simulink model "Simulation_traj"  (R2023a)
settings: Solver=FixedStepAuto  StartTime=0.0  StopTime=30  FixedStep=0.001  RelTol=1e-1
settings Model: Creator=mattia  LastModifiedBy=mattia
settings OptimizationCC: BlockReduction=off  DefaultParameterBehavior=Inlined  BufferReuse=off

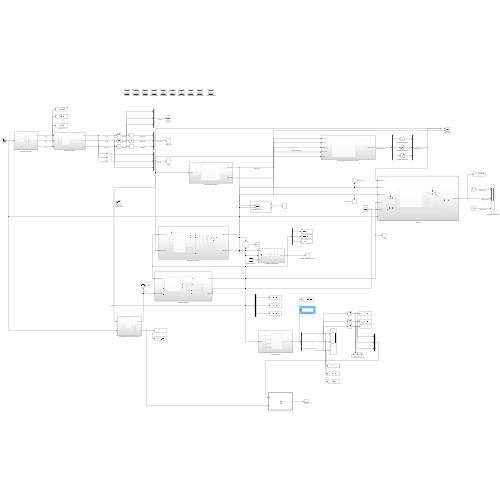
[thumbnail: Simulink's stored preview of the top-level diagram]
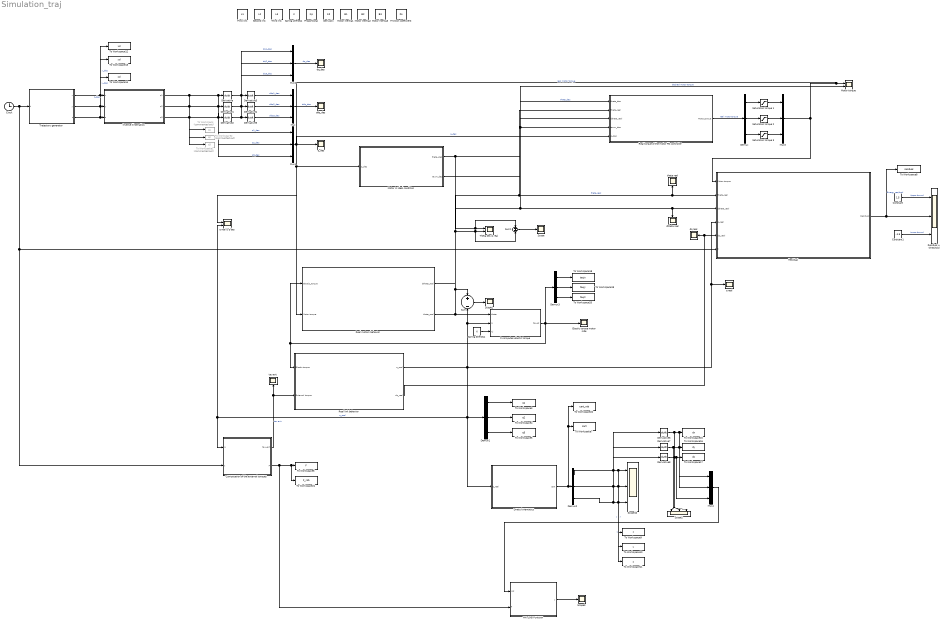
== system Simulation_traj ==
  Clock : Clock
  Computation of the external torques : Subsystem
  Constant : Constant  Value=1.5
  Constant1 : Constant  Value=-1.5
  Demux{,1..3} (4 alike) : Demux  Outputs=3
  Derivativ : DataStoreMemory  DataStoreName=Kd  WriteAfterWriteMsg=warning  InitialValue=50  ShowAdditionalParam=off
  Derivative{,1..8} (9 alike) : Derivative
  Direct kinematics : Subsystem
  Elastic torque motor side : Scope
  FIrst link : DataStoreMemory  DataStoreName=L1  WriteAfterWriteMsg=warning  InitialValue=0.5  ShowAdditionalParam=off
  Friction coefficient : DataStoreMemory  DataStoreName=Dv  WriteAfterWriteMsg=warning  InitialValue=0.8  ShowAdditionalParam=off
  Inverse Kinematics : Subsystem
  It computes elastic torque : Subsystem
  MATLAB Function : MATLAB Function  TreatAsAtomicUnit=on
  Motor Inertia1 : DataStoreMemory  DataStoreName=B1  WriteAfterWriteMsg=warning  InitialValue=0.45  ShowAdditionalParam=off
  Motor Inertia2 : DataStoreMemory  DataStoreName=B2  WriteAfterWriteMsg=warning  InitialValue=0.3037  ShowAdditionalParam=off
  Motor Inertia3 : DataStoreMemory  DataStoreName=B3  WriteAfterWriteMsg=warning  InitialValue=0.1199  ShowAdditionalParam=off
  Motor in ideal condition : Subsystem
  Motor torque : Scope  NumInputPorts=2
  Mux{,1..4} (5 alike) : Mux  Inputs=3
  Proportional : DataStoreMemory  DataStoreName=Kp  WriteAfterWriteMsg=warning  InitialValue=150  ShowAdditionalParam=off
  Real link behavior : Subsystem
  Real motors behavior : Subsystem
  Real torque of the motor PD controller : Subsystem
  Residual : Subsystem
  Residual + threshold : Scope  NumInputPorts=3
  Saturation torque 1 : Saturate  UpperLimit=80  LowerLimit=-80
  Saturation torque 2 : Saturate  UpperLimit=80  LowerLimit=-80
  Saturation torque 3 : Saturate  UpperLimit=80  LowerLimit=-80
  Scope : Scope
  Scope1 : Scope
  Scope10 : Scope  NumInputPorts=3
  Scope2 : Scope  NumInputPorts=3
  Scope3 : Scope
  Second link : DataStoreMemory  DataStoreName=L2  WriteAfterWriteMsg=warning  InitialValue=0.5  ShowAdditionalParam=off
  Spring Stiffness : DataStoreRead  DataStoreName=K  IndexOptions=Index vector (dialog)  Indices=1  OutputSizes=1
  Spring stiffness : DataStoreMemory  DataStoreName=K  WriteAfterWriteMsg=warning  InitialValue=9000  ShowAdditionalParam=off
  Sum : Sum  Inputs=+-
  Sum1 : Sum  Inputs=+-
  Theta des & real : Scope  NumInputPorts=2
  Third link : DataStoreMemory  DataStoreName=L3  WriteAfterWriteMsg=warning  InitialValue=0.4  ShowAdditionalParam=off
  To Workspace : ToWorkspace  Commented=on  VariableName=q1  SampleTime=-1
      settings: Save2DSignal=2-D array (concatenate along first dimension)
  To Workspace1 : ToWorkspace  Commented=on  VariableName=q3  SampleTime=-1
      settings: Save2DSignal=2-D array (concatenate along first dimension)
  To Workspace10 : ToWorkspace  VariableName=y
  To Workspace11 : ToWorkspace  VariableName=z
  To Workspace12 : ToWorkspace  VariableName=xd
  To Workspace13 : ToWorkspace  VariableName=yd
  To Workspace14 : ToWorkspace  VariableName=zd
  To Workspace15 : ToWorkspace  VariableName=dx
  To Workspace16 : ToWorkspace  VariableName=dy
  To Workspace17 : ToWorkspace  VariableName=dz
  To Workspace18 : ToWorkspace  VariableName=taujx
  To Workspace19 : ToWorkspace  VariableName=taujy
  To Workspace2 : ToWorkspace  Commented=on  VariableName=q2  SampleTime=-1
      settings: Save2DSignal=2-D array (concatenate along first dimension)
  To Workspace20 : ToWorkspace  VariableName=taujz
  To Workspace21 : ToWorkspace  VariableName=F_rob  SampleTime=0.3
  To Workspace22 : ToWorkspace  VariableName=cart_rob  SampleTime=0.3
  To Workspace3 : ToWorkspace  VariableName=q1  SampleTime=0.3
  To Workspace4 : ToWorkspace  VariableName=q2  SampleTime=0.3
  To Workspace5 : ToWorkspace  VariableName=q3  SampleTime=0.3
  To Workspace6 : ToWorkspace  VariableName=F  SampleTime=0.3
  To Workspace7 : ToWorkspace  VariableName=cart  SampleTime=0.3
  To Workspace8 : ToWorkspace  VariableName=residual
  To Workspace9 : ToWorkspace  VariableName=x
  Trajectory generator : Subsystem
  ddq_des : Scope
  dq real : Scope
  dq_des : Scope
  dtheta real : Scope
  q real : Scope
  q real & q des : Scope  NumInputPorts=2
  q_des : Scope
  tau ext : Scope
  theta real : Scope
  wires:
  Clock/1 -> Residual/6(t), Computation of the external torques/2(t), Trajectory generator/1(t)
  Trajectory generator/1(x) -> To Workspace12/1, Inverse Kinematics/1(x)  "x_des"
  Trajectory generator/2(y) -> To Workspace13/1, Inverse Kinematics/2(y)  "y_des"
  Trajectory generator/3(z) -> To Workspace14/1, Inverse Kinematics/3(z)  "z_des"
  Inverse Kinematics/1(q1) -> Derivative/1, Mux1/1, To Workspace/1  "q1_des"
  Inverse Kinematics/2(q2) -> Derivative1/1, Mux1/2, To Workspace2/1  "q2_des"
  Inverse Kinematics/3(q3) -> Mux1/3, Derivative2/1, To Workspace1/1  "q3_des"
  Derivative/1 -> Mux2/1, Derivative3/1  "dq1_des"
  Derivative1/1 -> Mux2/2, Derivative4/1  "dq2_des"
  Derivative2/1 -> Mux2/3, Derivative5/1  "dq3_des"
  Derivative3/1 -> Mux/1  "ddq1_des"
  Derivative4/1 -> Mux/2  "ddq2_des"
  Derivative5/1 -> Mux/3  "ddq3_des"
  Mux1/1 -> q_des/1, Real torque of the motor PD controller/5(q_des), Motor in ideal condition/1(q_des), q real & q des/1  "q_des"
  Mux/1 -> ddq_des/1  "ddq_des"
  Mux2/1 -> dq_des/1  "dq_des"
  Motor in ideal condition/2(taum_des) -> Real torque of the motor PD controller/4(taum_des), Motor torque/2  "desired motor torque"
  Motor in ideal condition/1(theta_des) -> Theta des & real/1, Sum1/1, Real torque of the motor PD controller/1(theta_des)  "theta_des"
  Real torque of the motor PD controller/1(Motor_torque) -> Demux/1  "real motor torque"
  Real motors behavior/2(theta_real) -> Residual/2(theta_real), theta real/1, Real torque of the motor PD controller/2(theta_real), Theta des & real/2, Sum1/2, Sum/1, It computes elastic torque/1(theta)  "theta_real"
  Real link behavior/1(q_real) -> Demux1/1, Direct kinematics/1(q_real), Computation of the external torques/1(q), q real & q des/2, Residual/4(q_real), q real/1, It computes elastic torque/2(q), Sum/2  "q_real"
  Real motors behavior/1(dtheta_real) -> Real torque of the motor PD controller/3(dtheta_real), dtheta real/1, Residual/3(dtheta_real)
  Demux1/2 -> To Workspace4/1
  Demux1/3 -> To Workspace5/1
  Real link behavior/2(dq_real) -> Residual/5(dq_real), dq real/1
  Residual/1(Residual) -> Residual + threshold/2, To Workspace8/1  "Energy residual"
  Computation of the external torques/1(tau_ext) -> tau ext/1, Real link behavior/2(External torque)  "tau ext"
  Demux/3 -> Saturation torque 3/1
  Saturation torque 2/1 -> Mux3/2
  Demux/2 -> Saturation torque 2/1
  Saturation torque 3/1 -> Mux3/3
  Demux/1 -> Saturation torque 1/1
  Saturation torque 1/1 -> Mux3/1
  Demux1/1 -> To Workspace3/1
  Direct kinematics/1(cart) -> To Workspace7/1, To Workspace22/1, Demux2/1
  Demux2/1 -> Derivative6/1, To Workspace9/1, Scope10/1  "x"
  Demux2/2 -> Derivative7/1, Scope10/2, To Workspace10/1  "y"
  Demux2/3 -> Scope10/3, To Workspace11/1, Derivative8/1  "z"
  Mux3/1 -> Real motors behavior/2(Motor torque), Motor torque/1, Residual/1(Motor torque)  "real motor torque"
  Sum1/1 -> Scope/1
  Spring Stiffness/1 -> It computes elastic torque/3(Kj)
  It computes elastic torque/1(tau_el) -> Demux3/1, Elastic torque motor side/1, Real link behavior/1(Elastic torque), Real motors behavior/1(Elastic_torque)
  Sum/1 -> Scope1/1
  Constant/1 -> Residual + threshold/1  "Upper bound"
  Constant1/1 -> Residual + threshold/3  "Lower bound"
  Computation of the external torques/2(F) -> MATLAB Function/2(F), To Workspace21/1, To Workspace6/1
  Derivative6/1 -> Mux4/1, To Workspace15/1, Scope2/1
  Derivative7/1 -> Scope2/3, Mux4/2, To Workspace16/1
  Derivative8/1 -> Mux4/3, To Workspace17/1, Scope2/2
  Mux4/1 -> MATLAB Function/1(vel)
  MATLAB Function/1(y) -> Scope3/1
  Demux3/1 -> To Workspace18/1
  Demux3/3 -> To Workspace20/1
  Demux3/2 -> To Workspace19/1

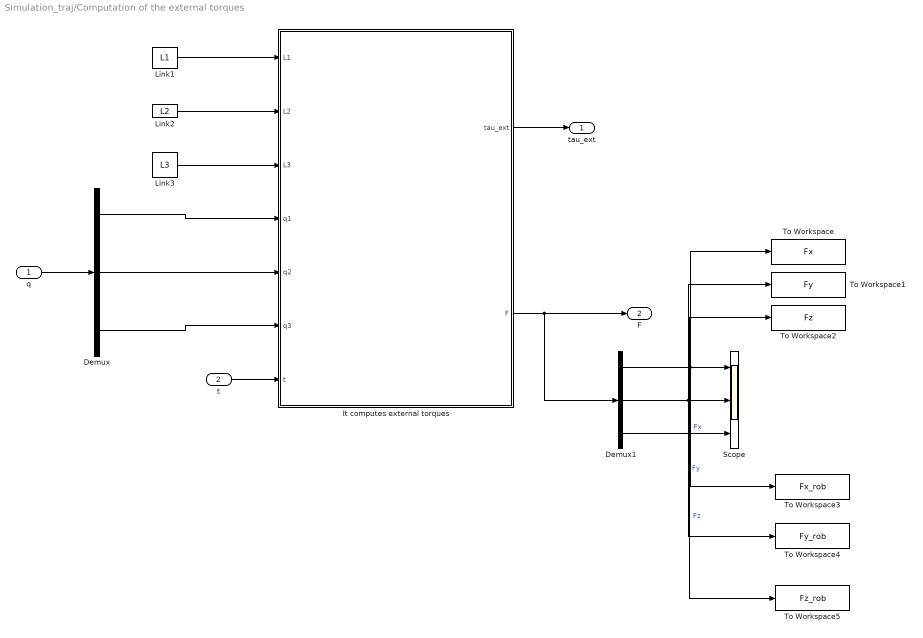
== system Simulation_traj/Computation of the external torques ==
  q : Inport
  t : Inport  Port=2
  Demux : Demux  Outputs=3
  Demux1 : Demux  Outputs=3
  It computes external torques : MATLAB Function  TreatAsAtomicUnit=on
  Link1 : DataStoreRead  DataStoreName=L1  IndexOptions=Index vector (dialog)  Indices=1  OutputSizes=1
  Link2 : DataStoreRead  DataStoreName=L2  IndexOptions=Index vector (dialog)  Indices=1  OutputSizes=1
  Link3 : DataStoreRead  DataStoreName=L3  IndexOptions=Index vector (dialog)  Indices=1  OutputSizes=1
  Scope : Scope  NumInputPorts=3
  To Workspace : ToWorkspace  VariableName=Fx
  To Workspace1 : ToWorkspace  VariableName=Fy
  To Workspace2 : ToWorkspace  VariableName=Fz
  To Workspace3 : ToWorkspace  VariableName=Fx_rob  SaveFormat=Timeseries  SampleTime=0.3
  To Workspace4 : ToWorkspace  VariableName=Fy_rob  SaveFormat=Timeseries  SampleTime=0.3
  To Workspace5 : ToWorkspace  VariableName=Fz_rob  SaveFormat=Timeseries  SampleTime=0.3
  tau_ext : Outport
  F : Outport  Port=2
  wires:
  t/1 -> It computes external torques/7(t)
  It computes external torques/1(tau_ext) -> tau_ext/1
  Link3/1 -> It computes external torques/3(L3)
  Link2/1 -> It computes external torques/2(L2)
  It computes external torques/2(F) -> F/1, Demux1/1
  Link1/1 -> It computes external torques/1(L1)
  Demux/1 -> It computes external torques/4(q1)
  Demux/2 -> It computes external torques/5(q2)
  Demux/3 -> It computes external torques/6(q3)
  q/1 -> Demux/1
  Demux1/2 -> Scope/2, To Workspace4/1, To Workspace1/1  "Fy"
  Demux1/1 -> Scope/1, To Workspace3/1, To Workspace/1  "Fx"
  Demux1/3 -> Scope/3, To Workspace2/1, To Workspace5/1  "Fz"

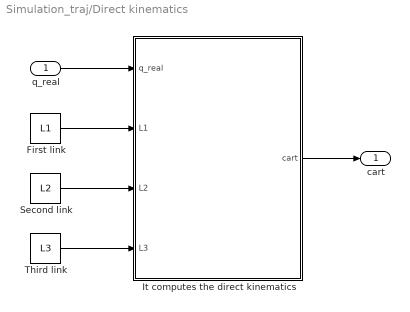
== system Simulation_traj/Direct kinematics ==
  q_real : Inport
  First link : DataStoreRead  DataStoreName=L1  IndexOptions=Index vector (dialog)  Indices=1  OutputSizes=1
  It computes the direct kinematics : MATLAB Function  TreatAsAtomicUnit=on
  Second link : DataStoreRead  DataStoreName=L2  IndexOptions=Index vector (dialog)  Indices=1  OutputSizes=1
  Third link : DataStoreRead  DataStoreName=L3  IndexOptions=Index vector (dialog)  Indices=1  OutputSizes=1
  cart : Outport
  wires:
  q_real/1 -> It computes the direct kinematics/1(q_real)
  First link/1 -> It computes the direct kinematics/2(L1)
  It computes the direct kinematics/1(cart) -> cart/1
  Third link/1 -> It computes the direct kinematics/4(L3)
  Second link/1 -> It computes the direct kinematics/3(L2)

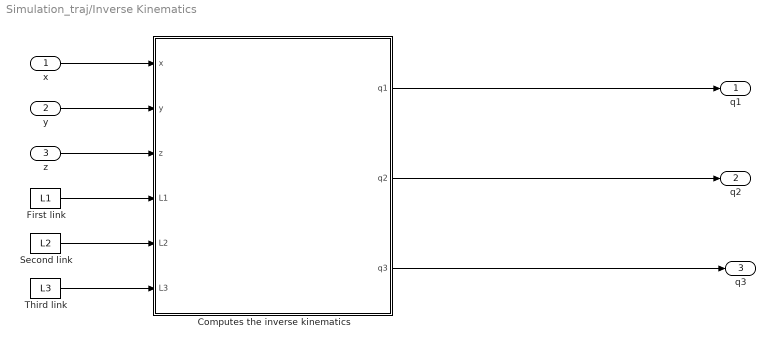
== system Simulation_traj/Inverse Kinematics ==
  x : Inport
  y : Inport  Port=2
  z : Inport  Port=3
  Computes the inverse kinematics : MATLAB Function  TreatAsAtomicUnit=on
  First link : DataStoreRead  DataStoreName=L1  IndexOptions=Index vector (dialog)  Indices=1  OutputSizes=1
  Second link : DataStoreRead  DataStoreName=L2  IndexOptions=Index vector (dialog)  Indices=1  OutputSizes=1
  Third link : DataStoreRead  DataStoreName=L3  IndexOptions=Index vector (dialog)  Indices=1  OutputSizes=1
  q1 : Outport
  q2 : Outport  Port=2
  q3 : Outport  Port=3
  wires:
  x/1 -> Computes the inverse kinematics/1(x)
  y/1 -> Computes the inverse kinematics/2(y)
  z/1 -> Computes the inverse kinematics/3(z)
  Computes the inverse kinematics/1(q1) -> q1/1
  Computes the inverse kinematics/2(q2) -> q2/1
  Computes the inverse kinematics/3(q3) -> q3/1
  First link/1 -> Computes the inverse kinematics/4(L1)
  Third link/1 -> Computes the inverse kinematics/6(L3)
  Second link/1 -> Computes the inverse kinematics/5(L2)

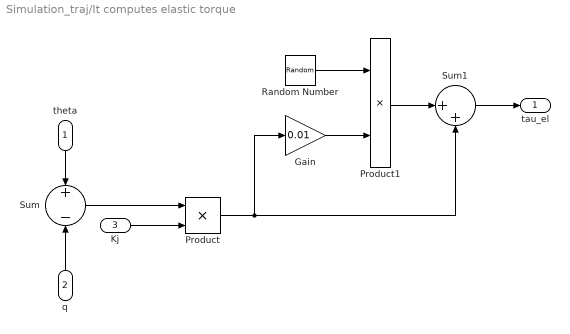
== system Simulation_traj/It computes elastic torque ==
  theta : Inport
  q : Inport  Port=2
  Kj : Inport  Port=3
  Gain : Gain  Gain=0.01
  Product : Product
  Product1 : Product
  Random Number : RandomNumber  SampleTime=0.1
  Sum : Sum  Inputs=+-
  Sum1 : Sum  Inputs=|++
  tau_el : Outport
  wires:
  q/1 -> Sum/2
  theta/1 -> Sum/1
  Sum/1 -> Product/1
  Kj/1 -> Product/2
  Product/1 -> Sum1/2, Gain/1
  Gain/1 -> Product1/2
  Random Number/1 -> Product1/1
  Product1/1 -> Sum1/1
  Sum1/1 -> tau_el/1

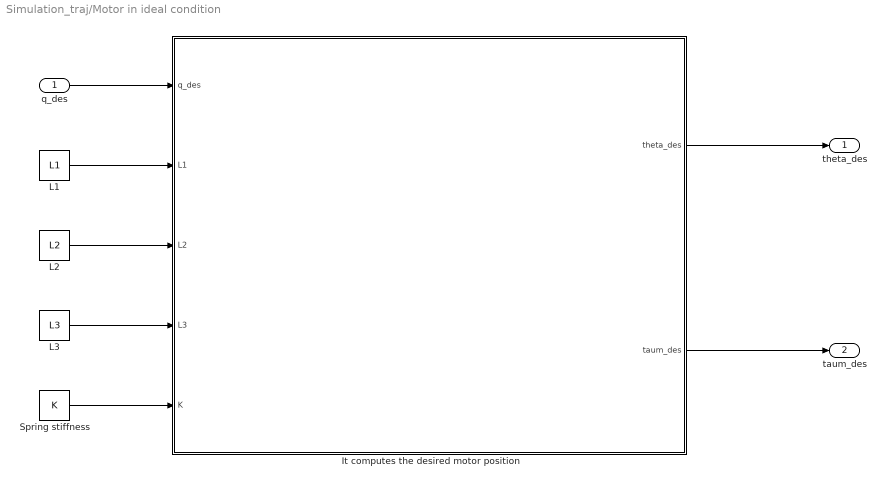
== system Simulation_traj/Motor in ideal condition ==
  q_des : Inport
  It computes the desired motor position : MATLAB Function  TreatAsAtomicUnit=on
  L1 : DataStoreRead  DataStoreName=L1  IndexOptions=Index vector (dialog)  Indices=1  OutputSizes=1
  L2 : DataStoreRead  DataStoreName=L2  IndexOptions=Index vector (dialog)  Indices=1  OutputSizes=1
  L3 : DataStoreRead  DataStoreName=L3  IndexOptions=Index vector (dialog)  Indices=1  OutputSizes=1
  Spring stiffness : DataStoreRead  DataStoreName=K  IndexOptions=Index vector (dialog)  Indices=1  OutputSizes=1
  theta_des : Outport
  taum_des : Outport  Port=2
  wires:
  L2/1 -> It computes the desired motor position/3(L2)
  It computes the desired motor position/1(theta_des) -> theta_des/1
  Spring stiffness/1 -> It computes the desired motor position/5(K)
  L3/1 -> It computes the desired motor position/4(L3)
  L1/1 -> It computes the desired motor position/2(L1)
  q_des/1 -> It computes the desired motor position/1(q_des)
  It computes the desired motor position/2(taum_des) -> taum_des/1

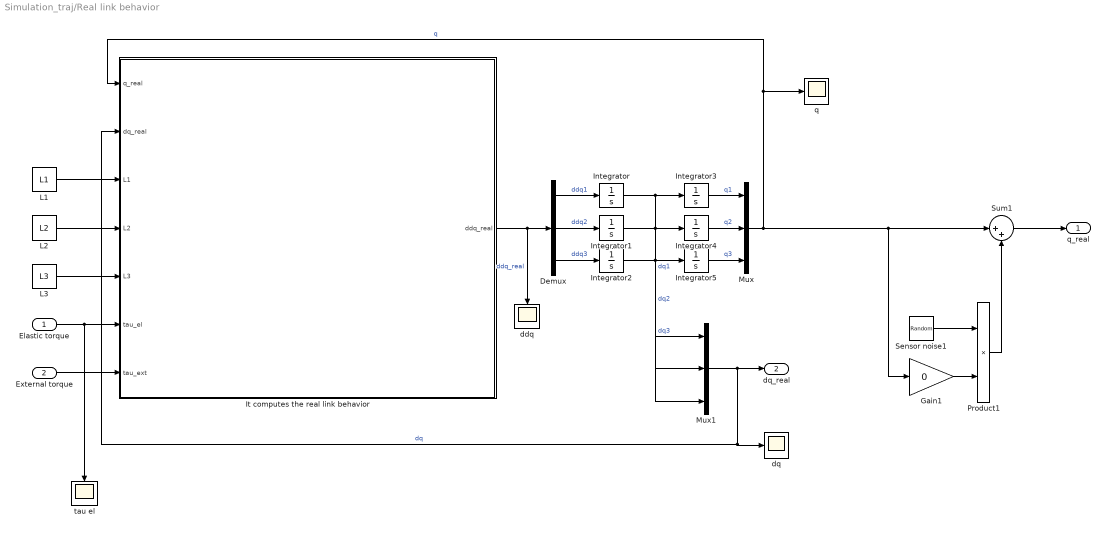
== system Simulation_traj/Real link behavior ==
  Elastic torque : Inport
  External torque : Inport  Port=2
  Demux : Demux  Outputs=3
  Gain1 : Gain  Gain=0
  Integrator : Integrator
  Integrator1 : Integrator
  Integrator2 : Integrator
  Integrator3 : Integrator  InitialCondition=1.6
  Integrator4 : Integrator  InitialCondition=-0.75
  Integrator5 : Integrator  InitialCondition=2
  It computes the real link behavior : MATLAB Function  TreatAsAtomicUnit=on
  L1 : DataStoreRead  DataStoreName=L1  IndexOptions=Index vector (dialog)  Indices=1  OutputSizes=1
  L2 : DataStoreRead  DataStoreName=L2  IndexOptions=Index vector (dialog)  Indices=1  OutputSizes=1
  L3 : DataStoreRead  DataStoreName=L3  IndexOptions=Index vector (dialog)  Indices=1  OutputSizes=1
  Mux : Mux  Inputs=3
  Mux1 : Mux  Inputs=3
  Product1 : Product
  Sensor noise1 : RandomNumber  SampleTime=0.1
  Sum1 : Sum  Inputs=|++
  ddq : Scope
  dq : Scope
  q : Scope
  tau el : Scope
  q_real : Outport
  dq_real : Outport  Port=2
  wires:
  It computes the real link behavior/1(ddq_real) -> Demux/1, ddq/1  "ddq_real"
  L1/1 -> It computes the real link behavior/3(L1)
  L2/1 -> It computes the real link behavior/4(L2)
  L3/1 -> It computes the real link behavior/5(L3)
  Demux/1 -> Integrator/1  "ddq1"
  Integrator/1 -> Integrator3/1, Mux1/1  "dq1"
  Demux/2 -> Integrator1/1  "ddq2"
  Demux/3 -> Integrator2/1  "ddq3"
  Integrator1/1 -> Integrator4/1, Mux1/2  "dq2"
  Integrator2/1 -> Integrator5/1, Mux1/3  "dq3"
  Integrator3/1 -> Mux/1  "q1"
  Integrator4/1 -> Mux/2  "q2"
  Integrator5/1 -> Mux/3  "q3"
  Mux/1 -> Sum1/1, Gain1/1, It computes the real link behavior/1(q_real), q/1  "q"
  Mux1/1 -> dq_real/1, dq/1, It computes the real link behavior/2(dq_real)  "dq"
  Elastic torque/1 -> It computes the real link behavior/6(tau_el), tau el/1
  External torque/1 -> It computes the real link behavior/7(tau_ext)
  Sensor noise1/1 -> Product1/1
  Gain1/1 -> Product1/2
  Product1/1 -> Sum1/2
  Sum1/1 -> q_real/1

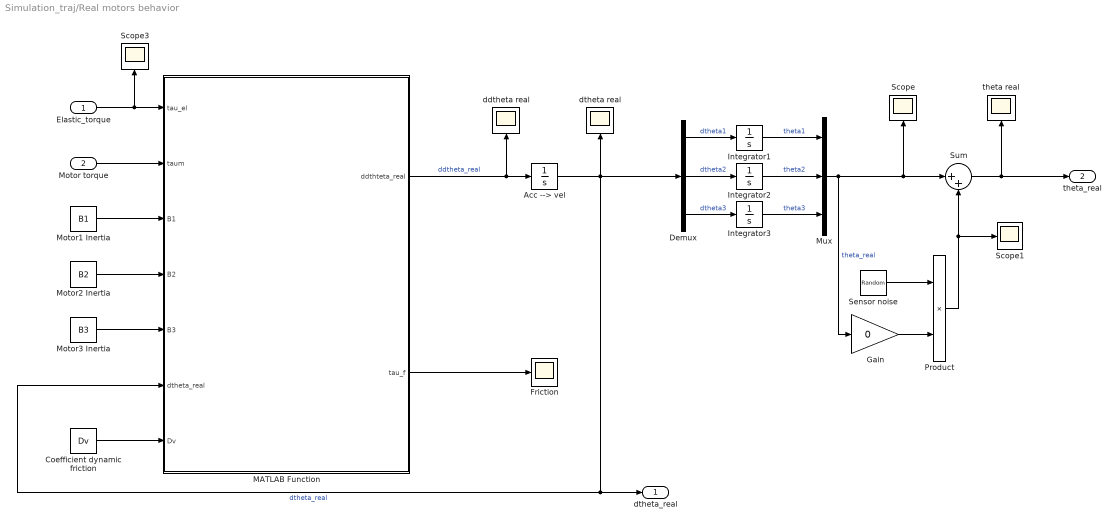
== system Simulation_traj/Real motors behavior ==
  Elastic_torque : Inport
  Motor torque : Inport  Port=2
  Acc --> vel : Integrator  InitialCondition=0.01
  Coefficient dynamic friction : DataStoreRead  DataStoreName=Dv  IndexOptions=Index vector (dialog)  Indices=1  OutputSizes=1
  Demux : Demux  Outputs=3
  Friction : Scope
  Gain : Gain  Gain=0
  Integrator1 : Integrator  InitialCondition=1.6
  Integrator2 : Integrator  InitialCondition=-0.75
  Integrator3 : Integrator  InitialCondition=2
  MATLAB Function : MATLAB Function  TreatAsAtomicUnit=on
  Motor1 Inertia : DataStoreRead  DataStoreName=B1  IndexOptions=Index vector (dialog)  Indices=1  OutputSizes=1
  Motor2 Inertia : DataStoreRead  DataStoreName=B2  IndexOptions=Index vector (dialog)  Indices=1  OutputSizes=1
  Motor3 Inertia : DataStoreRead  DataStoreName=B3  IndexOptions=Index vector (dialog)  Indices=1  OutputSizes=1
  Mux : Mux  Inputs=3
  Product : Product
  Scope : Scope
  Scope1 : Scope
  Scope3 : Scope
  Sensor noise : RandomNumber  SampleTime=0.1
  Sum : Sum  Inputs=|++
  ddtheta real : Scope
  dtheta real : Scope
  theta real : Scope
  dtheta_real : Outport
  theta_real : Outport  Port=2
  wires:
  Elastic_torque/1 -> MATLAB Function/1(tau_el), Scope3/1
  Motor1 Inertia/1 -> MATLAB Function/3(B1)
  Acc --> vel/1 -> Demux/1, dtheta_real/1, MATLAB Function/6(dtheta_real), dtheta real/1  "dtheta_real"
  Coefficient dynamic friction/1 -> MATLAB Function/7(Dv)
  Motor torque/1 -> MATLAB Function/2(taum)
  Demux/1 -> Integrator1/1  "dtheta1"
  Demux/2 -> Integrator2/1  "dtheta2"
  Demux/3 -> Integrator3/1  "dtheta3"
  Integrator1/1 -> Mux/1  "theta1"
  Integrator2/1 -> Mux/2  "theta2"
  Integrator3/1 -> Mux/3  "theta3"
  Mux/1 -> Sum/1, Scope/1, Gain/1  "theta_real"
  Motor2 Inertia/1 -> MATLAB Function/4(B2)
  Motor3 Inertia/1 -> MATLAB Function/5(B3)
  MATLAB Function/2(tau_f) -> Friction/1
  MATLAB Function/1(ddthteta_real) -> Acc --> vel/1, ddtheta real/1  "ddtheta_real"
  Sum/1 -> theta_real/1, theta real/1
  Sensor noise/1 -> Product/1
  Gain/1 -> Product/2
  Product/1 -> Scope1/1, Sum/2

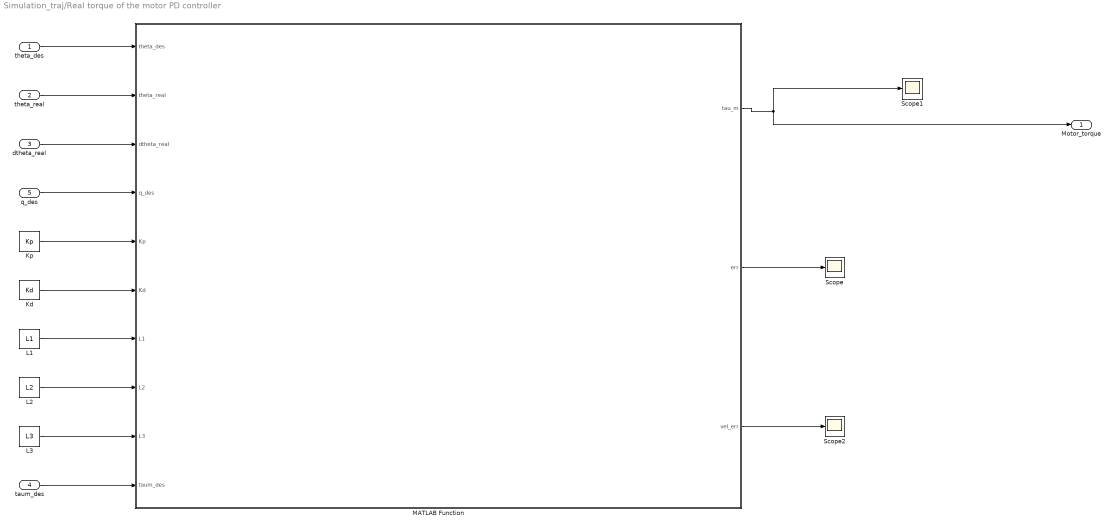
== system Simulation_traj/Real torque of the motor PD controller ==
  theta_des : Inport
  theta_real : Inport  Port=2
  dtheta_real : Inport  Port=3
  taum_des : Inport  Port=4
  q_des : Inport  Port=5
  Kd : DataStoreRead  DataStoreName=Kd  IndexOptions=Index vector (dialog)  Indices=1  OutputSizes=1
  Kp : DataStoreRead  DataStoreName=Kp  IndexOptions=Index vector (dialog)  Indices=1  OutputSizes=1
  L1 : DataStoreRead  DataStoreName=L1  IndexOptions=Index vector (dialog)  Indices=1  OutputSizes=1
  L2 : DataStoreRead  DataStoreName=L2  IndexOptions=Index vector (dialog)  Indices=1  OutputSizes=1
  L3 : DataStoreRead  DataStoreName=L3  IndexOptions=Index vector (dialog)  Indices=1  OutputSizes=1
  MATLAB Function : MATLAB Function  TreatAsAtomicUnit=on
  Scope : Scope
  Scope1 : Scope
  Scope2 : Scope
  Motor_torque : Outport
  wires:
  theta_des/1 -> MATLAB Function/1(theta_des)
  theta_real/1 -> MATLAB Function/2(theta_real)
  dtheta_real/1 -> MATLAB Function/3(dtheta_real)
  q_des/1 -> MATLAB Function/4(q_des)
  Kp/1 -> MATLAB Function/5(Kp)
  Kd/1 -> MATLAB Function/6(Kd)
  L1/1 -> MATLAB Function/7(L1)
  L2/1 -> MATLAB Function/8(L2)
  L3/1 -> MATLAB Function/9(L3)
  taum_des/1 -> MATLAB Function/10(taum_des)
  MATLAB Function/1(tau_m) -> Motor_torque/1, Scope1/1
  MATLAB Function/2(err) -> Scope/1
  MATLAB Function/3(vel_err) -> Scope2/1

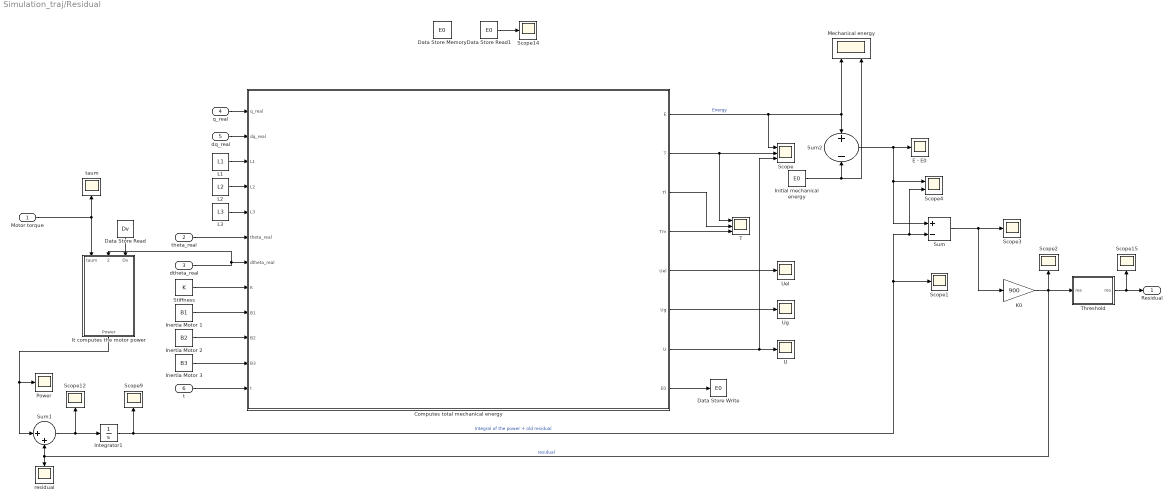
== system Simulation_traj/Residual ==
  Motor torque : Inport
  theta_real : Inport  Port=2
  dtheta_real : Inport  Port=3
  q_real : Inport  Port=4
  dq_real : Inport  Port=5
  t : Inport  Port=6
  Computes total mechanical energy : MATLAB Function  TreatAsAtomicUnit=on
  Data Store Memory : DataStoreMemory  DataStoreName=E0  WriteAfterWriteMsg=warning  ShowAdditionalParam=off
  Data Store Read : DataStoreRead  DataStoreName=Dv  IndexOptions=Index vector (dialog)  Indices=1  OutputSizes=1
  Data Store Read1 : DataStoreRead  DataStoreName=E0  IndexOptions=Index vector (dialog)  Indices=1  OutputSizes=1
  Data Store Write : DataStoreWrite  DataStoreName=E0  IndexOptions=Index vector (dialog)  Indices=1  OutputSizes=1
  E - E0 : Scope
  Inertia Motor 1 : DataStoreRead  DataStoreName=B1  IndexOptions=Index vector (dialog)  Indices=1  OutputSizes=1
  Inertia Motor 2 : DataStoreRead  DataStoreName=B2  IndexOptions=Index vector (dialog)  Indices=1  OutputSizes=1
  Inertia Motor 3 : DataStoreRead  DataStoreName=B3  IndexOptions=Index vector (dialog)  Indices=1  OutputSizes=1
  Initial mechanical energy : DataStoreRead  DataStoreName=E0  IndexOptions=Index vector (dialog)  Indices=1  OutputSizes=1
  Integrator1 : Integrator
  It computes the motor power : MATLAB Function  TreatAsAtomicUnit=on
  K0 : Gain  Gain=900
  L1 : DataStoreRead  DataStoreName=L1  IndexOptions=Index vector (dialog)  Indices=1  OutputSizes=1
  L2 : DataStoreRead  DataStoreName=L2  IndexOptions=Index vector (dialog)  Indices=1  OutputSizes=1
  L3 : DataStoreRead  DataStoreName=L3  IndexOptions=Index vector (dialog)  Indices=1  OutputSizes=1
  Mechanical energy : Scope  NumInputPorts=2
  Power : Scope
  Scope : Scope  NumInputPorts=3
  Scope{1..3,9,12,14..15} (7 alike) : Scope
  Scope4 : Scope  NumInputPorts=2
  Stiffness : DataStoreRead  DataStoreName=K  IndexOptions=Index vector (dialog)  Indices=1  OutputSizes=1
  Sum : Sum  Inputs=+-
  Sum1 : Sum  Inputs=|++
  Sum2 : Sum  Inputs=+-
  T : Scope  NumInputPorts=3
  Threshold : MATLAB Function  TreatAsAtomicUnit=on
  U : Scope
  Uel : Scope
  Ug : Scope
  residual : Scope
  taum : Scope
  Residual : Outport
  wires:
  Sum/1 -> Scope3/1, K0/1
  Integrator1/1 -> Scope9/1, Sum/2, Scope4/2, Scope1/1  "Integral of the power + old residual"
  It computes the motor power/1(Power) -> Sum1/1, Power/1
  Sum1/1 -> Integrator1/1, Scope12/1
  Computes total mechanical energy/1(E) -> Mechanical energy/1, Sum2/1, Scope/1  "Energy"
  K0/1 -> Sum1/2, residual/1, Scope2/1, Threshold/1("res ")  "residual"
  L3/1 -> Computes total mechanical energy/5(L3)
  Stiffness/1 -> Computes total mechanical energy/8(K)
  L1/1 -> Computes total mechanical energy/3(L1)
  L2/1 -> Computes total mechanical energy/4(L2)
  dtheta_real/1 -> It computes the motor power/2(dtheta_real), Computes total mechanical energy/7(dtheta_real)
  Inertia Motor 1/1 -> Computes total mechanical energy/9(B1)
  q_real/1 -> Computes total mechanical energy/1(q_real)
  dq_real/1 -> Computes total mechanical energy/2(dq_real)
  theta_real/1 -> Computes total mechanical energy/6(theta_real)
  Threshold/1(res) -> Residual/1, Scope15/1
  Data Store Read/1 -> It computes the motor power/3(Dv)
  Motor torque/1 -> It computes the motor power/1(taum), taum/1
  Inertia Motor 2/1 -> Computes total mechanical energy/10(B2)
  Inertia Motor 3/1 -> Computes total mechanical energy/11(B3)
  Data Store Read1/1 -> Scope14/1
  Computes total mechanical energy/2(T) -> Scope/2, T/1
  Computes total mechanical energy/7(U) -> Scope/3, U/1
  Computes total mechanical energy/3(Tl) -> T/2
  Computes total mechanical energy/5(Uel) -> Uel/1
  Computes total mechanical energy/6(Ug) -> Ug/1
  Computes total mechanical energy/8(E0) -> Data Store Write/1
  Initial mechanical energy/1 -> Sum2/2, Mechanical energy/2
  Sum2/1 -> E - E0/1, Sum/1, Scope4/1
  t/1 -> Computes total mechanical energy/12(t)
  Computes total mechanical energy/4(Tm) -> T/3

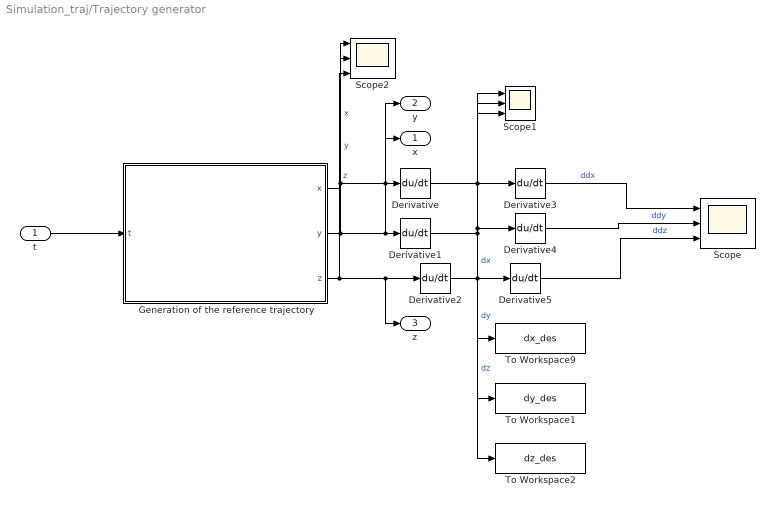
== system Simulation_traj/Trajectory generator ==
  t : Inport
  Derivative{,1..5} (6 alike) : Derivative
  Generation of the reference trajectory : MATLAB Function  TreatAsAtomicUnit=on
  Scope : Scope  NumInputPorts=3
  Scope1 : Scope  NumInputPorts=3
  Scope2 : Scope  NumInputPorts=3
  To Workspace1 : ToWorkspace  VariableName=dy_des
  To Workspace2 : ToWorkspace  VariableName=dz_des
  To Workspace9 : ToWorkspace  VariableName=dx_des
  x : Outport
  y : Outport  Port=2
  z : Outport  Port=3
  wires:
  Derivative/1 -> To Workspace9/1, Scope1/1, Derivative3/1  "dx"
  Derivative1/1 -> Scope1/2, Derivative4/1, To Workspace1/1  "dy"
  Derivative2/1 -> Scope1/3, Derivative5/1, To Workspace2/1  "dz"
  t/1 -> Generation of the reference trajectory/1(t)
  Generation of the reference trajectory/1(x) -> Scope2/1, x/1, Derivative/1  "x"
  Generation of the reference trajectory/3(z) -> Scope2/3, z/1, Derivative2/1  "z"
  Generation of the reference trajectory/2(y) -> Scope2/2, y/1, Derivative1/1  "y"
  Derivative3/1 -> Scope/1  "ddx"
  Derivative4/1 -> Scope/2  "ddy"
  Derivative5/1 -> Scope/3  "ddz"

== matlab function Simulation_traj/Residual/It computes the motor power ==
  data: taum input; dtheta_real input; Power output; Dv input
function Power = power(taum, dtheta_real, Dv)
Dv = diag([Dv Dv Dv]);
Power = dtheta_real'*(taum + Dv*dtheta_real);

== matlab function Simulation_traj/Motor in ideal condition/It computes the desired motor position ==
  data: q_des input; L1 input; theta_des output; L2 input; L3 input; K input; taum_des output
function [theta_des, taum_des] = desired_motor_position(q_des, L1, L2,L3, K)

dc1=L1/2; % link CoMs (on local x axis) [m]
dc2=L2/2; 
dc3=L3/2;

m1=15; % link masses [kg]
m2=10;
m3=5;
g0 = 9.81; 

q1 = q_des(1);
q2 = q_des(2);
q3 = q_des(3);

G =   [0
       g0*m3*(dc3*cos(q2 + q3) + L2*cos(q2)) + dc2*g0*m2*cos(q2)
       dc3*g0*m3*cos(q2 + q3)];

K = diag([K, K, K]);

theta_des = q_des + inv(K)*G;
taum_des = G;

== matlab function Simulation_traj/Real torque of the motor PD controller/MATLAB Function ==
  data: theta_des input; tau_m output; theta_real input; dtheta_real input; q_des input; Kp input; Kd input; L1 input; L2 input; L3 input; taum_des input; err output; vel_err output
function [tau_m, err, vel_err]  = tau_motor(theta_des, theta_real, dtheta_real, q_des, Kp, Kd, L1, L2, L3, taum_des)


dc1=L1/2; % link CoMs (on local x axis) [m]
dc2=L2/2; 
dc3=L3/2;

m1=15; % link masses [kg]
m2=10;
m3=5;
g0 = 9.81; 

q1 = q_des(1);
q2 = q_des(2);
q3 = q_des(3);

G =   [0
       g0*m3*(dc3*cos(q2 + q3) + L2*cos(q2)) + dc2*g0*m2*cos(q2)
       dc3*g0*m3*cos(q2 + q3)];

Kp = diag([Kp Kp Kp]);
Kd = diag([Kd Kd Kd]); 


tau_m = Kp*(theta_des - theta_real) - Kd*dtheta_real + taum_des;
err = Kp*(theta_des - theta_real);
vel_err = -dtheta_real;

== matlab function Simulation_traj/Real motors behavior/MATLAB Function ==
  data: tau_el input; ddthteta_real output; taum input; B1 input; B2 input; B3 input; dtheta_real input; Dv input; tau_f output
function [ddthteta_real, tau_f] = real_motor_position(tau_el, taum, B1, B2, B3, dtheta_real, Dv)

B = diag([B1 B2 B3]);
ddthteta_real = [0;0;0];
Dv = diag([Dv Dv Dv]);
tau_f = -Dv*dtheta_real;
ddthteta_real = inv(B)*(taum - tau_el + tau_f);

== matlab function Simulation_traj/Computation of the external torques/It computes external torques ==
  data: L1 input; tau_ext output; L2 input; L3 input; q1 input; q2 input; q3 input; t input; F output
function [tau_ext, F] = compute_external_torque(L1, L2, L3, q1, q2, q3, t)

tau_ext = [0;0;0];

F = [0;0;0];
J_ee = [ -sin(q1)*(L3*cos(q2 + q3) + L2*cos(q2)),  -cos(q1)*(L3*sin(q2 + q3) + L2*sin(q2)),  -L3*sin(q2 + q3)*cos(q1)
          cos(q1)*(L3*cos(q2 + q3) + L2*cos(q2)),  -sin(q1)*(L3*sin(q2 + q3) + L2*sin(q2)),  -L3*sin(q2 + q3)*sin(q1)
                                              0,              L3*cos(q2 + q3) + L2*cos(q2),           L3*cos(q2 + q3)];

J_third_joint = [ -sin(q1)*L2*cos(q2),           -cos(q1)*L2*sin(q2),         0
                   cos(q1)*L2*cos(q2),            -sin(q1)*L2*sin(q2),         0
                                   0,            L2*cos(q2),                  0];
l2 = 0.35;
l3 = 0.2;

J_third_link = [-sin(q1)*(l3*cos(q2 + q3) + L2*cos(q2)), -cos(q1)*(l3*sin(q2 + q3) + L2*sin(q2)),      -l3*sin(q2 + q3)*cos(q1)
                cos(q1)*(l3*cos(q2 + q3) + L2*cos(q2)),  -sin(q1)*(l3*sin(q2 + q3) + L2*sin(q2)),      -l3*sin(q2 + q3)*sin(q1)
                                      0,                 l3*cos(q2 + q3) + L2*cos(q2),                 l3*cos(q2 + q3)];

J_second_link = [-sin(q1)*l2*cos(q2),                  -cos(q1)*l2*sin(q2),         0
                 cos(q1)*l2*cos(q2),                   -sin(q1)*l2*sin(q2),         0
                                      0,               l2*cos(q2),                  0];
J_fake = [ -sin(q1)*(L3*cos(q2 + q3) + L2*cos(q2)),  -cos(q1)*(L3*sin(q2 + q3) + L2*sin(q2)),  0
          cos(q1)*(L3*cos(q2 + q3) + L2*cos(q2)),  -sin(q1)*(L3*sin(q2 + q3) + L2*sin(q2)),  0
                                              0,              L3*cos(q2 + q3) + L2*cos(q2),           0];



if t > 3 && t < 6
    F = [-30; -20; 0];
    tau_ext = J_ee'*F;
end

if t > 12 && t < 16
    F = [0; 0; -15]; 
    tau_ext = J_third_link'*F;
end

if t > 18 && t < 23
    F_bis = [10; -20; 0];
    F = F_bis*(t-18)*0.5;
    tau_ext = J_ee'*F;
end

if t > 26 && t < 29
    F = [0; 0; -35];
    tau_ext = J_second_link'*F;
end

== matlab function Simulation_traj/Residual/Threshold ==
  data: res input; res output
function res = threshold(res)
threshold = 0;
if res > threshold || res < -threshold
    res = res;
else
    res = 0;
end

== matlab function Simulation_traj/Direct kinematics/It computes the direct kinematics ==
  data: q_real input; cart output; L1 input; L2 input; L3 input
function cart = direct_kin(q_real, L1, L2, L3)

q1 = q_real(1);
q2 = q_real(2);
q3 = q_real(3);

px = cos(q1)*(L2*cos(q2) + L3*cos(q2+q3));
py = sin(q1)*(L2*cos(q2) + L3*cos(q2+q3));
pz = L1 + L2*sin(q2) +L3*sin(q2+q3);

cart = [px; py; pz];

== matlab function Simulation_traj/MATLAB Function ==
  data: vel input; F input; y output
function y = fcn(vel, F)

y = F'*vel;

== matlab function Simulation_traj/Residual/Computes total mechanical energy ==
  data: q_real input; E output; T output; Tl output; Tm output; Uel output; Ug output; U output; dq_real input; L1 input; L2 input; L3 input; theta_real input; dtheta_real input; K input; B1 input; B2 input; B3 input; E0 output; t input
function [E, T, Tl, Tm, Uel, Ug, U, E0] = Mechanical_energy(q_real, dq_real, L1, L2, L3,  theta_real, dtheta_real,K, B1, B2, B3, t)
persistent initial_energy;
% Link energy
q1 = q_real(1);
q2 = q_real(2);
q3 = q_real(3);

dq1 = dq_real(1);
dq2 = dq_real(2);
dq3 = dq_real(3);

dc1=L1/2; % link CoMs (on local x axis) [m]
dc2=L2/2; 
dc3=L3/2; 

m1=15; % link masses [kg]
m2=10;
m3=5;

r1=0.2;  % links as full cylinders with uniform mass of radius r [m] 
I1zz=(1/2)*m1*r1^2; % [kg*m^2]
r2=0.1;
I2xx=(1/2)*m2*r2^2;
I2yy=(1/12)*m2*(3*r2^2+L2^2);
I2zz=I2yy;
r3=0.1;
I3xx=(1/2)*m3*r3^2;
I3yy=(1/12)*m3*(3*r3^2+L3^2);
I3zz=I3yy;
g0=9.81; % acceleration of gravity [m/s^2]

T1 = (I1zz*dq1^2)/2;
T2 = (I2yy*dq2^2)/2 + (I2yy*dq1^2*cos(q2)^2)/2 + (I2xx*dq1^2*sin(q2)^2)/2 + (dc2^2*m2*(dq1^2 - dq1^2*sin(q2)^2 + dq2^2))/2;
T3 = (I3xx*dq1^2)/4 + (I3yy*dq1^2)/4 + (I3yy*dq2^2)/2 + (I3yy*dq3^2)/2 + (L2^2*dq1^2*m3)/4 + (L2^2*dq2^2*m3)/2 + (dc3^2*dq1^2*m3)/4 + (dc3^2*dq2^2*m3)/2 + (dc3^2*dq3^2*m3)/2 + I3yy*dq2*dq3 - (I3xx*dq1^2*cos(2*q2 + 2*q3))/4 + (I3yy*dq1^2*cos(2*q2 + 2*q3))/4 + dc3^2*dq2*dq3*m3 + (L2^2*dq1^2*m3*cos(2*q2))/4 + (dc3^2*dq1^2*m3*cos(2*q2 + 2*q3))/4 + (L2*dc3*dq1^2*m3*cos(q3))/2 + L2*dc3*dq2^2*m3*cos(q3) + (L2*dc3*dq1^2*m3*cos(2*q2 + q3))/2 + L2*dc3*dq2*dq3*m3*cos(q3);

Tl = T1 + T2 + T3;

U1 = 0;
U2 = g0*m2*(L1 + dc2*sin(q2));
U3 = g0*m3*(L1 + dc3*sin(q2 + q3) + L2*sin(q2));

Ug = U1 + U2 + U3;

% Motor energy

B = diag([B1, B2, B3]);

Tm = 1/2*dtheta_real'*B*dtheta_real; % Kinetic energy of the motors

Kj = diag([K K K]);
Uel = 1/2*(theta_real - q_real)'*Kj*(theta_real - q_real); % elastic energy due to the elastic coupling of the joints

T = Tl + Tm;
U = Ug + Uel;

E = T + U;
if isempty(initial_energy)
    initial_energy = T + U;
end
E0 = initial_energy;

== matlab function Simulation_traj/Trajectory generator/Generation of the reference trajectory ==
  data: x output; t input; y output; z output
function [x, y, z] = Trajectory_generation(t)
r = 0.3;            % Circle radius
w = pi / 9;         % Angular velocity
x = 0;
y = 0;
z = 0;
x_0 = -0.3;          % Circle center X coordinate
y_0 = 0.5;          % Circle center Y coordinate
z_0 = 0.5;          % Circle center Z coordinate
T1 = 10;
T2 = 20;
T3 = 30;

if t >= 0 && t <= T1
    theta = w * t;
    x = x_0 + r * cos(theta);
    y = y_0; 
    z = z_0 + r * sin(theta);
end

if t >= T1 && t <= T2
    theta = w * T1;
    x = x_0 + r * cos(theta);
    y = y_0;
    z = z_0 + r * sin(theta);
end

if t >= T2 && t <= T3
    theta = w * T1;
    x = x_0 + r*cos(theta) - 0.1 * (t - T2) / (T3 - T2);
    y = y_0 - 0.4* (t - T2) / (T3 - T2);
    z = z_0 + r*sin(theta);
end

== matlab function Simulation_traj/Real link behavior/It computes the real link behavior ==
  data: q_real input; ddq_real output; dq_real input; L1 input; L2 input; L3 input; tau_el input; tau_ext input
function ddq_real  = real_links(q_real, dq_real, L1, L2, L3, tau_el, tau_ext)
ddq_real = [0;0;0];
dc1=L1/2; % link CoMs (on local x axis) [m]
dc2=L2/2; 
dc3=L3/2;

m1=15; % link masses [kg]
m2=10;
m3=5;

r1=0.2;  % links as full cylinders with uniform mass of radius r [m] 
I1zz=(1/2)*m1*r1^2; % [kg*m^2]
r2=0.1;
I2xx=(1/2)*m2*r2^2;
I2yy=(1/12)*m2*(3*r2^2+L2^2);
I2zz=I2yy;
r3=0.1;
I3xx=(1/2)*m3*r3^2;
I3yy=(1/12)*m3*(3*r3^2+L3^2);
I3zz=I3yy;

g0=9.81; % acceleration of gravity [m/s^2]

q1 = q_real(1);
q2 = q_real(2);
q3 = q_real(3);

dq1 = dq_real(1);
dq2 = dq_real(2);
dq3 = dq_real(3);

M = [I3xx/2 + I3yy/2 + I1zz - (I3xx*cos(2*q2 + 2*q3))/2 + (I3yy*cos(2*q2 + 2*q3))/2 + (L2^2*m3)/2 + (dc3^2*m3)/2 + I2yy*cos(q2)^2 + I2xx*sin(q2)^2 - (dc2^2*m2*(2*sin(q2)^2 - 2))/2 + (L2^2*m3*cos(2*q2))/2 + (dc3^2*m3*cos(2*q2 + 2*q3))/2 + L2*dc3*m3*cos(q3) + L2*dc3*m3*cos(2*q2 + q3),                                                                 0,                                   0;
                                                                                                                                                                                                                                                                                    0, m3*L2^2 + 2*m3*cos(q3)*L2*dc3 + m2*dc2^2 + m3*dc3^2 + I2yy + I3yy, m3*dc3^2 + L2*m3*cos(q3)*dc3 + I3yy;
                                                                                                                                                                                                                                                                                   0,                               m3*dc3^2 + L2*m3*cos(q3)*dc3 + I3yy,                     m3*dc3^2 + I3yy];
a1=I1zz+I2xx+I3xx;
a2=I2yy+m2*dc2^2+m3*L2^2-I2xx;
a3=I3yy+m3*dc3^2-I3xx;
a4=m3*L2*dc3;
a5=I2yy+m2*dc2^2+m3*dc3^2+I3yy+m3*L2^2;
a6=I3yy+m3*dc3^2;

c = [- dq1*(dq2*(a4*sin(2*q2 + q3) + a3*cos(q2 + q3)*sin(q2 + q3) + a2*cos(q2)*sin(q2)) + dq3*((a4*sin(q3))/2 + (a4*sin(2*q2 + q3))/2 + a3*cos(q2 + q3)*sin(q2 + q3))) - dq1*dq3*((a4*sin(q3))/2 + (a4*sin(2*q2 + q3))/2 + a3*cos(q2 + q3)*sin(q2 + q3)) - dq1*dq2*(a4*sin(2*q2 + q3) + a3*cos(q2 + q3)*sin(q2 + q3) + a2*cos(q2)*sin(q2));
     (a4*sin(2*q2 + q3) + a3*cos(q2 + q3)*sin(q2 + q3) + a2*cos(q2)*sin(q2))*dq1^2 - dq3*(a4*dq2*sin(q3) + a4*dq3*sin(q3)) - a4*dq2*dq3*sin(q3);
     ((a4*sin(q3))/2 + (a4*sin(2*q2 + q3))/2 + a3*cos(q2 + q3)*sin(q2 + q3))*dq1^2 + a4*sin(q3)*dq2^2];  

G =   [0
       g0*m3*(dc3*cos(q2 + q3) + L2*cos(q2)) + dc2*g0*m2*cos(q2)
       dc3*g0*m3*cos(q2 + q3)];

ddq_real = inv(M)*(tau_el + tau_ext - c - G);

== matlab function Simulation_traj/Inverse Kinematics/Computes the inverse kinematics ==
  data: x input; q1 output; y input; z input; q2 output; q3 output; L1 input; L2 input; L3 input
function [q1,q2,q3] = Inverse_kinematics(x, y, z, L1, L2, L3)

c3 = (x^2 + y^2 + (z - L1)^2 - L2^2 - L3^2)/(2*L2*L3);
s3 = sqrt(1 - c3^2);
q3 = atan2(s3,c3);
% if q3 < 0
%     q3 = q3 + 2*pi;
% end

q1 = atan2(y,x);
% if q1 < 0
%     q1 = q1 + 2*pi;
% end
c1 = cos(q1);
s1 = sin(q1);

A = [L2 + L3*c3 -L3*s3; L3*s3 L2 + L3*c3];
b = [c1*x + s1*y; z - L1];
sol = inv(A)*b;
c2 = sol(1);
s2 = sol(2);

q2 = atan2(s2,c2);
% if q2 < 0
%     q2 = q2 + 2*pi;
% end
end
